simulink model "modelTest"  (R2025a)
settings: Solver=VariableStepAuto  StartTime=0.0  StopTime=1000  MaxStep=0.001  RelTol=1e-3
libraries: simulink x6
settings Model: Creator=levirogalla  LastModifiedBy=levirogalla

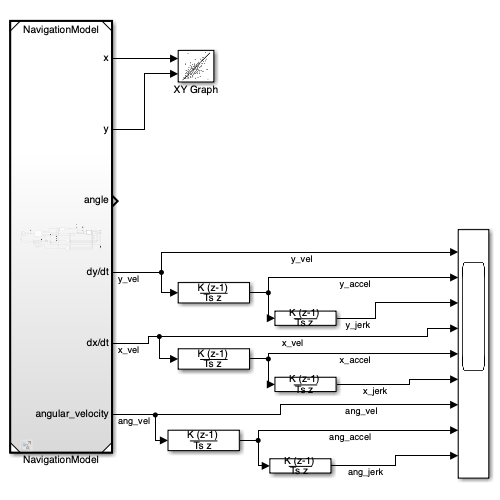
[thumbnail: Simulink's stored preview of the top-level diagram]
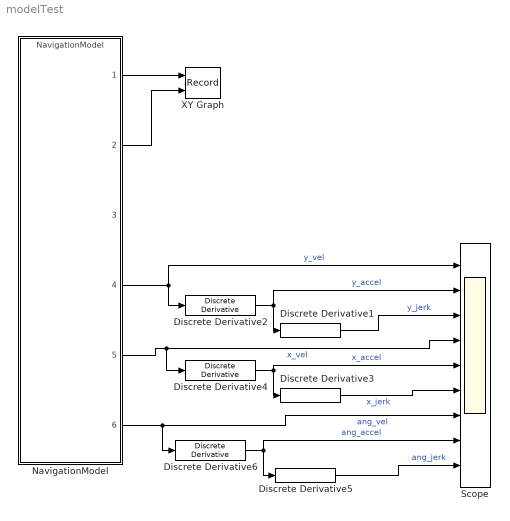
== system modelTest ==
  Discrete Derivative{1..6} (6 alike) : simulink/Discrete/Discrete Derivative  gainval=1.0  ICPrevScaledInput=0.0  OutMin=[]  OutMax=[]  OutDataType=fixdt(1, 16)  OutScaling=2^-10  DoSatur=off
  NavigationModel : ModelReference  ModelNameDialog=NavigationModel.slx  SimulationMode=Normal  ModelReferenceVersion=1.99
  Scope : Scope  NumInputPorts=9
      settings: ActiveDisplayYMinimum=-0.34288942513811804  ActiveDisplayYMaximum=0.36422591548751232
  XY Graph : Record  NumPorts=2.0  FileSettingsInternal="{\"entries\":[{\"content\":{\"excelSettings\":{\"content\":{},\"type\":\"Streamout.ExcelSettings\"},\"parquetSettings\":{\"content\":{},\"type\":\"Streamout.ParquetSettings\"}},\"type\":\"Streamout.FileSettingStorage\",\"uuid\":\"\"}],\"packageUris\":[\"http:\\/\\/schema.mathworks.com\\/mf0\\/streamout_blocks\\/R2020a\"],\"version\":\"1.0\"}"  FrameSettings=[0, 0]  Layout=[1 1]  SignalsInternal="{\"entries\":[{\"content\":{\"signals\":[{\"content\":{\"blockPath\":[],\"dimensions\":[1],\"domain\":\"\",\"lineColor\":\"#a2142f\",\"plots\":[ 1 ],\"port\":1,\"sid\":[\"\"],\"signalID\":1,\"signalName\":\"NavigationModel:1\"},\"type\":\"RecordBlkView.Signal\",\"uuid\":\"\"},{\"content\":{\"blockPath\":[],\"dimensions\":[1],\"domain\":\"\",\"lineColor\":\"#139fff\",\"plots\":[ 1 ],\"port\":2,\"sid\":[\"\"],\"signalID\":2,\"signalName\":\"NavigationModel:2\"},\"type\":\"RecordBlkView.Signal\",\"uuid\":\"\"}]},\"type\":\"RecordBlkView.InputSignals\",\"uuid\":\"\"}],\"packageUris\":[\"http:\\/\\/schema.mathworks.com\\/mf0\\/streamout_blocks\\/R2020a\"],\"version\":\"1.0\"}"  VisualizationBindings="{\"xyplotplugin\":{\"info\":[{\"series\":[{\"bindingParametersList\":[{\"parameter\":\"X-Axis\",\"signalID\":1,\"signalName\":\"NavigationModel:1\"},{\"parameter\":\"Y-Axis\",\"signalID\":2,\"signalName\":\"NavigationModel:2\"}],\"seriesID\":0}],\"subplotID\":1}]}}"  CompatibilityTag=XY
  wires:
  NavigationModel/1 -> XY Graph/1
  NavigationModel/2 -> XY Graph/2
  NavigationModel/4 -> Scope/1, Discrete Derivative2/1  "y_vel"
  Discrete Derivative2/1 -> Discrete Derivative1/1, Scope/2  "y_accel"
  Discrete Derivative4/1 -> Discrete Derivative3/1, Scope/5  "x_accel"
  Discrete Derivative6/1 -> Scope/8, Discrete Derivative5/1  "ang_accel"
  Discrete Derivative1/1 -> Scope/3  "y_jerk"
  NavigationModel/5 -> Discrete Derivative4/1, Scope/4  "x_vel"
  Discrete Derivative3/1 -> Scope/6  "x_jerk"
  NavigationModel/6 -> Discrete Derivative6/1, Scope/7  "ang_vel"
  Discrete Derivative5/1 -> Scope/9  "ang_jerk"
